simulink model "dcmotorpowerlibrary"  (R2024b)
settings: Solver=VariableStepAuto  StartTime=0.0  StopTime=200  RelTol=1e-3
libraries: spsDCMachineLib x1, simulink x1, spsControlledVoltageSourceLib x1, spsDCVoltageSourceLib x1, sps_lib x1
settings Model: Creator=brain  LastModifiedBy=brain

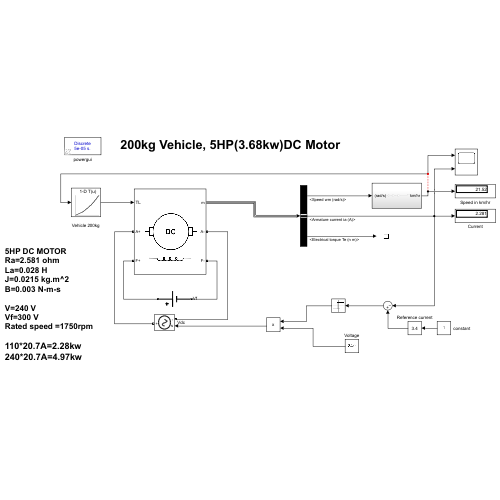
[thumbnail: Simulink's stored preview of the top-level diagram]
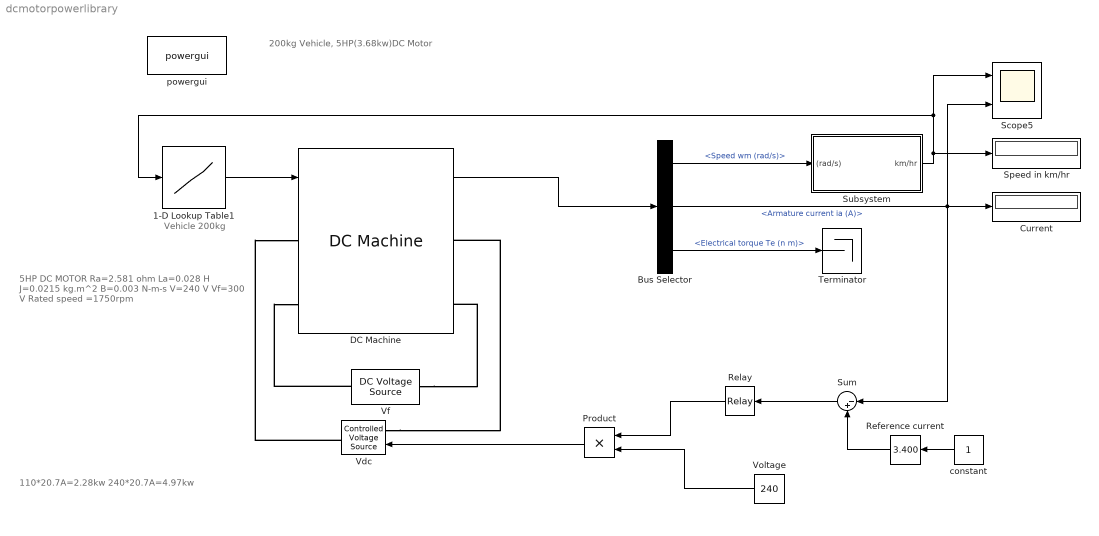
== system dcmotorpowerlibrary ==
  note: 110*20.7A=2.28kw
      | 240*20.7A=4.97kw
  note: Vehicle 200kg
  note: 200kg Vehicle, 5HP(3.68kw)DC Motor
  note: 5HP DC MOTOR
      | Ra=2.581 ohm
      | La=0.028 H
      | J=0.0215 kg.m^2
      | B=0.003 N-m-s
      |
      | V=240 V
      | Vf=300 V
      | Rated speed =1750rpm
  1-D Lookup Table1 : Lookup_n-D  NumberOfTableDimensions=1  BreakpointsForDimension1=[28.4 56.8 63.5 69.56 75.13 80.32 85.19 89.8 94.19 98.37 102.4 106.3 110 113.6 117.1 120.5 123.8 127]  Table=[5 20 25 30 35 40 45 50 55 60 65 70 75 80 85 90 95 100]  InternalRulePriority=Speed  RndMeth=Simplest
  Bus Selector : BusSelector  OutputSignals=Speed wm (rad/s),Armature current ia (A),Electrical torque Te (n m)
  Current : Display
  DC Machine : spsDCMachineLib/DC Machine  PresetModel=No  MechanicalLoad=Torque TL  FieldType=Wound  ShowDetailedParameters=on  MeasurementBus=off  RLa="[ 02.581  0.028]"  RLf="[ 281.3  3.156]"  Laf=0.9483  MachineConstant=Torque constant (N.m/A)  Ke=1.8  Kt=1.8  J=200*0.279*0.279  Bm=0.002953  Tf=0.5161  w0=1  Ifinit=1.06647707074298  TsPowergui=0  TsBlock=-1
  Product : Product
  Reference current : simulink/Math Operations/Slider Gain  gain=3.400  low=1  high=21
  Relay : Relay  OnSwitchValue=1  OffSwitchValue=-1
  Scope5 : Scope  NumInputPorts=2
  Speed in km/hr : Display
  Subsystem : Subsystem
  Sum : Sum  Inputs=|-+
  Terminator : Terminator
  Vdc : spsControlledVoltageSourceLib/Controlled Voltage Source  Initialize=on  Source_Type=DC  Amplitude=0  Phase=0  Frequency=0  Measurements=None
  Vf : spsDCVoltageSourceLib/DC Voltage Source  Amplitude=300  Measurements=None
  Voltage : Constant  Value=240
  constant : Constant
  powergui : sps_lib/powergui  Priority=1  SimulationMode=Discrete  SampleTime=50e-6  frequency=60  Iterations=50  frequencyindice=0  Pbase=100e6  ErrMax=1e-4  UnitsV=kV  UnitsW=MW  buscounter=0  FunctionMessages=off  echomessages=off  EnableUseOfTLC=off  CurrentSourceSwitches=off  DisableSnubberDevices=off  DisableRonSwitches=off  DisableVfSwitches=off  DisplayEquations=off  AutomaticDiscreteSolvers=off  SolverType=Tustin/Backward Euler (TBE)  Interpol=off  ExternalGateDelay=off  methode=off  Ts=100  x0status=blocks  SPID=on  SwTol=0  HookPort=off  NonlinearTolerance=1e-4  nMaxIteration=100  ContinueOnMaxIteration=off  RestoreLinks=warning  ResistiveCurrentMeasurement=off  Frange=[0:2:500]  Ylog=off  Xlog=on  ShowGrid=off  save=off  variable=ZData  structure=0  ZoomFFT=off  StartTime=0.0  cycles=1  DisplayStyle=1  fundamental=60  FreqAxis=off  MaxFrequency=1000  frequencyindicesteady=1  RmsSteady=1  display=off
  wires:
  DC Machine/1 -> Bus Selector/1
  1-D Lookup Table1/1 -> DC Machine/1
  Subsystem/1(km/hr) -> 1-D Lookup Table1/1, Scope5/1, Speed in km/hr/1
  Bus Selector/1 -> Subsystem/1(" (rad/s)")  "<Speed wm (rad/s)>"
  Bus Selector/2 -> Sum/1, Current/1, Scope5/2  "<Armature current ia (A)>"
  Bus Selector/3 -> Terminator/1  "<Electrical torque Te (n m)>"
  constant/1 -> Reference current/1
  Sum/1 -> Relay/1
  Relay/1 -> Product/1
  Voltage/1 -> Product/2
  Product/1 -> Vdc/1
  Reference current/1 -> Sum/2
  connections:
  Vf/RConn1 -- DC Machine/LConn2
  Vdc/RConn1 -- DC Machine/LConn1
  Vf/LConn1 -- DC Machine/RConn2
  Vdc/LConn1 -- DC Machine/RConn1

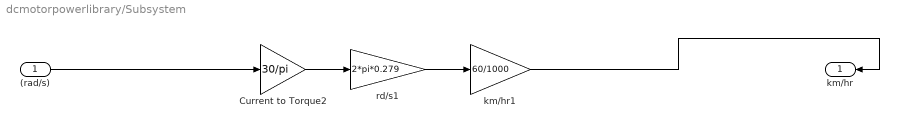
== system dcmotorpowerlibrary/Subsystem ==
  " (rad/s)" : Inport
  Current to Torque2 : Gain  Gain=30/pi
  km/hr1 : Gain  Gain=60/1000
  rd/s1 : Gain  Gain=2*pi*0.279
  km/hr : Outport
  wires:
  " (rad/s)"/1 -> Current to Torque2/1
  Current to Torque2/1 -> rd/s1/1
  rd/s1/1 -> km/hr1/1
  km/hr1/1 -> km/hr/1
